simulink model "Cinematica_inversa"  (R2022b)
settings: Solver=VariableStepAuto  StartTime=0.0  StopTime=10.0  RelTol=1e-3
settings Model: Creator=usuario  LastModifiedBy=usuario

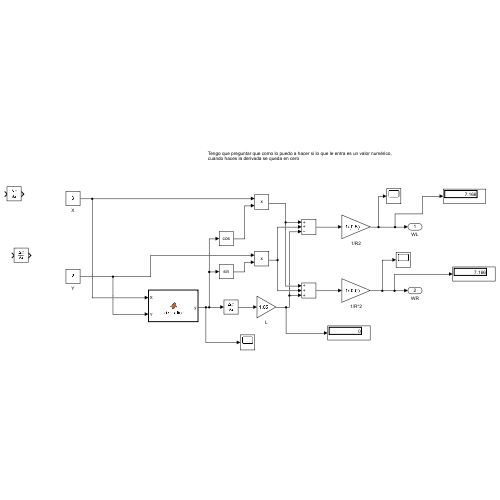
[thumbnail: Simulink's stored preview of the top-level diagram]
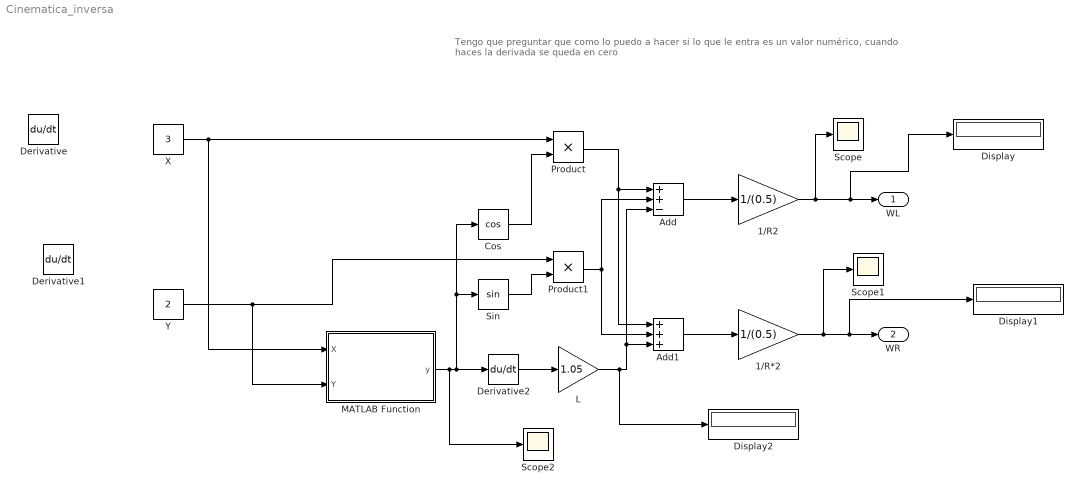
== system Cinematica_inversa ==
  note: Tengo que preguntar que como lo puedo a hacer si lo que le entra es un valor numérico, cuando haces la derivada se queda en cero
  1/R*2 : Gain  Gain=1/(0.5)
  1/R2 : Gain  Gain=1/(0.5)
  Add : Sum  Inputs=++-
  Add1 : Sum  Inputs=+++
  Cos : Trigonometry  Operator=cos
  Derivative : Derivative
  Derivative1 : Derivative
  Derivative2 : Derivative
  Display : Display
  Display1 : Display
  Display2 : Display
  L : Gain  Gain=1.05
  MATLAB Function : MATLAB Function  TreatAsAtomicUnit=on
  Product : Product
  Product1 : Product
  Scope : Scope
  Scope1 : Scope
  Scope2 : Scope
  Sin : Trigonometry
  X : Constant  Value=3
  Y : Constant  Value=2
  WL : Outport
  WR : Outport  Port=2
  wires:
  Cos/1 -> Product/2
  MATLAB Function/1(y) -> Scope2/1, Derivative2/1, Cos/1, Sin/1
  Sin/1 -> Product1/2
  Product/1 -> Add1/1, Add/1
  Product1/1 -> Add1/2, Add/2
  Derivative2/1 -> L/1
  L/1 -> Display2/1, Add/3, Add1/3
  Add/1 -> 1/R2/1
  Add1/1 -> 1/R*2/1
  1/R2/1 -> Scope/1, Display/1, WL/1
  1/R*2/1 -> Scope1/1, Display1/1, WR/1
  X/1 -> MATLAB Function/1(X), Product/1
  Y/1 -> MATLAB Function/2(Y), Product1/1

== matlab function Cinematica_inversa/MATLAB Function ==
  data: X input; y output; Y input
function y = orientation(X ,Y )

    R=0.5;
    L=1.05/2;

    O = (R/(2*L))*(X-Y);
   


y = O;
